simulink model "top_model"  (R2016a)
settings: Solver=ode1  StartTime=0  StopTime=20  FixedStep=0.001  RelTol=1e-3
undefined symbols (not defined in the file): env, veh_tyr, veh_veh_sx_0, veh_veh_vx_0
settings Model: Creator=The MathWorks, Inc.  LastModifiedBy=Renata
settings SolverCC: MaxOrder=3
settings DataIOCC: LimitDataPoints=on
settings DebuggingCC: AllowSymbolicDim=off
settings ModelReferenceCC: PropagateSignalLabelsOutOfModel=off
settings GRTTargetCC: GeneratePreprocessorConditionals=Use local settings

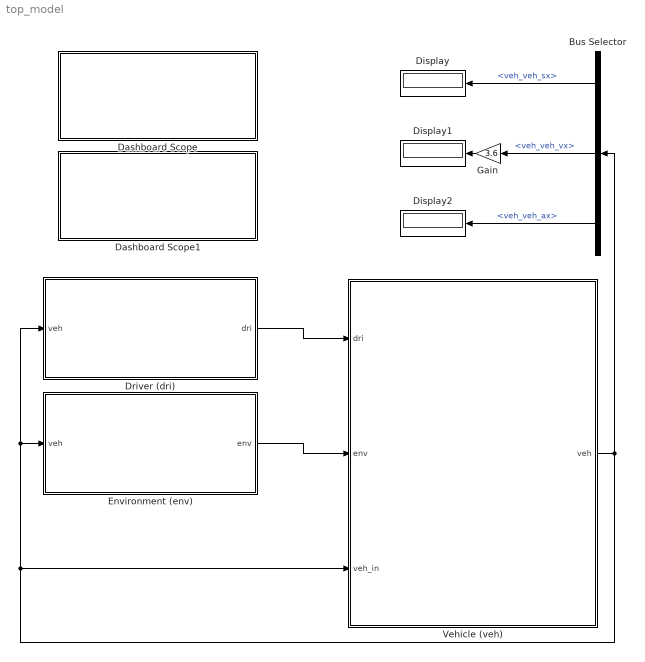
== system top_model ==
  Bus Selector : BusSelector  OutputSignals=veh_veh.veh_veh_sx,veh_veh.veh_veh_vx,veh_veh.veh_veh_ax
  Dashboard Scope : Subsystem  DialogController=hmiCreateDDGDialog  IsWebBlock=on  mask(MWDashboardBlock){webBlockId=2edd3ace-788d-40da-b228-b60fa6116b31, webBlockType=sdiscope, ShowInitialText=on, HMISrcModelName=top_model}
      mask prompts: webBlockId "WebBlock Id"; webBlockType "WebBlock Type"; HMISrcModelName "Source Model"
      mask Help: helpview([docroot '/mapfiles/simulink.map'], 'hmi_scope')
      mask Display:
      | if strcmp(get_param(bdroot(gcb),'BlockDiagramType'), 'library')
      |     image([(matlabroot) '/toolbox/simulink/hmi/icons/DashboardScope.png']);
      | end
  Dashboard Scope1 : Subsystem  DialogController=hmiCreateDDGDialog  IsWebBlock=on  mask(MWDashboardBlock){webBlockId=645ad2c4-08cc-4e51-8054-379eba2c8f07, webBlockType=sdiscope, ShowInitialText=on, HMISrcModelName=top_model}
      mask prompts: webBlockId "WebBlock Id"; webBlockType "WebBlock Type"; HMISrcModelName "Source Model"
      mask Help: helpview([docroot '/mapfiles/simulink.map'], 'hmi_scope')
      mask Display:
      | if strcmp(get_param(bdroot(gcb),'BlockDiagramType'), 'library')
      |     image([(matlabroot) '/toolbox/simulink/hmi/icons/DashboardScope.png']);
      | end
  Display : Display
  Display1 : Display
  Display2 : Display
  Driver (dri) : Subsystem  VariantControl=Variant
  Environment (env) : Subsystem
  Gain : Gain  Gain=3.6
  Vehicle (veh) : Subsystem
  wires:
  Driver (dri)/1(dri) -> Vehicle (veh)/1(dri)
  Environment (env)/1(env) -> Vehicle (veh)/2(env)
  Vehicle (veh)/1(veh) -> Bus Selector/1, Driver (dri)/1(veh), Environment (env)/1(veh), Vehicle (veh)/3(veh_in)
  Bus Selector/1 -> Display/1  "<veh_veh_sx>"
  Bus Selector/2 -> Gain/1  "<veh_veh_vx>"
  Bus Selector/3 -> Display2/1  "<veh_veh_ax>"
  Gain/1 -> Display1/1

== system top_model/Dashboard Scope ==

== system top_model/Dashboard Scope1 ==

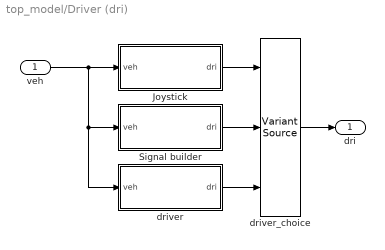
== system top_model/Driver (dri) ==
  veh : Inport
  Joystick : Subsystem  VariantControl=Variant
  Signal builder : Subsystem  VariantControl=Variant
  driver : Subsystem  VariantControl=Variant
  driver_choice : VariantSource  ShowConditionOnBlock=on
  dri : Outport
  wires:
  Signal builder/1(dri) -> driver_choice/2
  driver/1(dri) -> driver_choice/3
  Joystick/1(dri) -> driver_choice/1
  driver_choice/1 -> dri/1
  veh/1 -> driver/1(veh), Signal builder/1(veh), Joystick/1(veh)

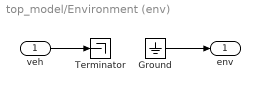
== system top_model/Environment (env) ==
  veh : Inport
  Ground : Ground
  Terminator : Terminator
  env : Outport
  wires:
  veh/1 -> Terminator/1
  Ground/1 -> env/1

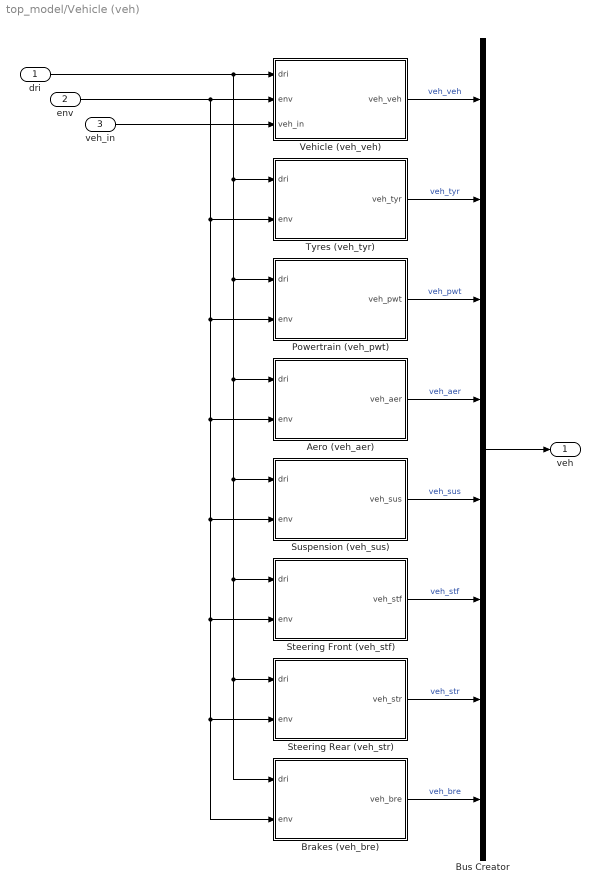
== system top_model/Vehicle (veh) ==
  dri : Inport
  env : Inport  Port=2
  veh_in : Inport  Port=3
  Aero (veh_aer) : Subsystem
  Brakes (veh_bre) : Subsystem
  Bus Creator : BusCreator  Inputs=8
  Powertrain (veh_pwt) : Subsystem
  Steering Front (veh_stf) : Subsystem
  Steering Rear (veh_str) : Subsystem
  Suspension (veh_sus) : Subsystem
  Tyres (veh_tyr) : Subsystem
  Vehicle (veh_veh) : Subsystem
  veh : Outport
  wires:
  Brakes (veh_bre)/1(veh_bre) -> Bus Creator/8  "veh_bre"
  Steering Rear (veh_str)/1(veh_str) -> Bus Creator/7  "veh_str"
  Steering Front (veh_stf)/1(veh_stf) -> Bus Creator/6  "veh_stf"
  Suspension (veh_sus)/1(veh_sus) -> Bus Creator/5  "veh_sus"
  Aero (veh_aer)/1(veh_aer) -> Bus Creator/4  "veh_aer"
  Powertrain (veh_pwt)/1(veh_pwt) -> Bus Creator/3  "veh_pwt"
  Tyres (veh_tyr)/1(veh_tyr) -> Bus Creator/2  "veh_tyr"
  Vehicle (veh_veh)/1(veh_veh) -> Bus Creator/1  "veh_veh"
  Bus Creator/1 -> veh/1
  dri/1 -> Brakes (veh_bre)/1(dri), Steering Rear (veh_str)/1(dri), Steering Front (veh_stf)/1(dri), Suspension (veh_sus)/1(dri), Aero (veh_aer)/1(dri), Powertrain (veh_pwt)/1(dri), Tyres (veh_tyr)/1(dri), Vehicle (veh_veh)/1(dri)
  env/1 -> Brakes (veh_bre)/2(env), Steering Rear (veh_str)/2(env), Steering Front (veh_stf)/2(env), Suspension (veh_sus)/2(env), Aero (veh_aer)/2(env), Powertrain (veh_pwt)/2(env), Tyres (veh_tyr)/2(env), Vehicle (veh_veh)/2(env)
  veh_in/1 -> Vehicle (veh_veh)/3(veh_in)

== system top_model/Driver (dri)/Joystick ==
  veh : Inport
  Ground : Ground
  Terminator : Terminator
  dri : Outport
  wires:
  veh/1 -> Terminator/1
  Ground/1 -> dri/1

== system top_model/Driver (dri)/Signal builder ==
  veh : Inport
  Ground : Ground
  Terminator : Terminator
  dri : Outport
  wires:
  veh/1 -> Terminator/1
  Ground/1 -> dri/1

== system top_model/Driver (dri)/driver ==
  veh : Inport
  Ground : Ground
  Terminator : Terminator
  dri : Outport
  wires:
  veh/1 -> Terminator/1
  Ground/1 -> dri/1

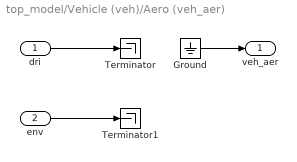
== system top_model/Vehicle (veh)/Aero (veh_aer) ==
  dri : Inport
  env : Inport  Port=2
  Ground : Ground
  Terminator : Terminator
  Terminator1 : Terminator
  veh_aer : Outport
  wires:
  dri/1 -> Terminator/1
  env/1 -> Terminator1/1
  Ground/1 -> veh_aer/1

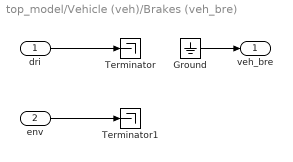
== system top_model/Vehicle (veh)/Brakes (veh_bre) ==
  dri : Inport
  env : Inport  Port=2
  Ground : Ground
  Terminator : Terminator
  Terminator1 : Terminator
  veh_bre : Outport
  wires:
  dri/1 -> Terminator/1
  env/1 -> Terminator1/1
  Ground/1 -> veh_bre/1

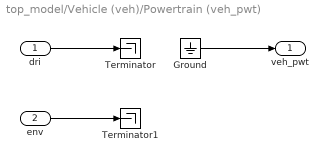
== system top_model/Vehicle (veh)/Powertrain (veh_pwt) ==
  dri : Inport
  env : Inport  Port=2
  Ground : Ground
  Terminator : Terminator
  Terminator1 : Terminator
  veh_pwt : Outport
  wires:
  dri/1 -> Terminator/1
  env/1 -> Terminator1/1
  Ground/1 -> veh_pwt/1

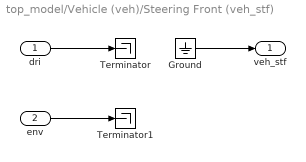
== system top_model/Vehicle (veh)/Steering Front (veh_stf) ==
  dri : Inport
  env : Inport  Port=2
  Ground : Ground
  Terminator : Terminator
  Terminator1 : Terminator
  veh_stf : Outport
  wires:
  dri/1 -> Terminator/1
  env/1 -> Terminator1/1
  Ground/1 -> veh_stf/1

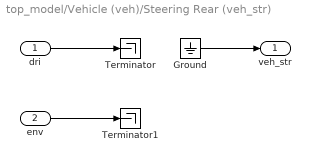
== system top_model/Vehicle (veh)/Steering Rear (veh_str) ==
  dri : Inport
  env : Inport  Port=2
  Ground : Ground
  Terminator : Terminator
  Terminator1 : Terminator
  veh_str : Outport
  wires:
  dri/1 -> Terminator/1
  env/1 -> Terminator1/1
  Ground/1 -> veh_str/1

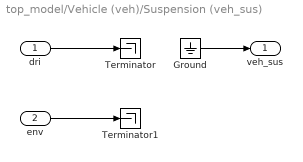
== system top_model/Vehicle (veh)/Suspension (veh_sus) ==
  dri : Inport
  env : Inport  Port=2
  Ground : Ground
  Terminator : Terminator
  Terminator1 : Terminator
  veh_sus : Outport
  wires:
  dri/1 -> Terminator/1
  env/1 -> Terminator1/1
  Ground/1 -> veh_sus/1

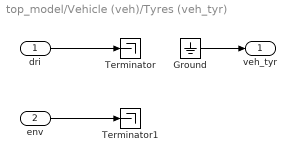
== system top_model/Vehicle (veh)/Tyres (veh_tyr) ==
  dri : Inport
  env : Inport  Port=2
  Ground : Ground
  Terminator : Terminator
  Terminator1 : Terminator
  veh_tyr : Outport
  wires:
  Ground/1 -> veh_tyr/1
  dri/1 -> Terminator/1
  env/1 -> Terminator1/1

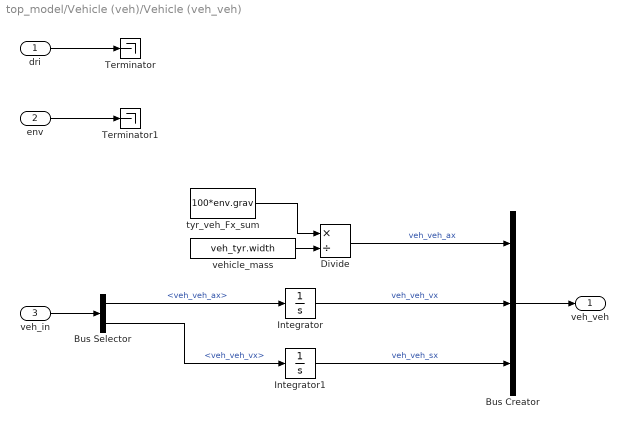
== system top_model/Vehicle (veh)/Vehicle (veh_veh) ==
  dri : Inport
  env : Inport  Port=2
  veh_in : Inport  Port=3
  Bus Creator : BusCreator  Inputs=3
  Bus Selector : BusSelector  OutputSignals=veh_veh.veh_veh_ax,veh_veh.veh_veh_vx
  Divide : Product  Inputs=*/  SaturateOnIntegerOverflow=on  RndMeth=Zero
  Integrator : Integrator  InitialCondition=veh_veh_vx_0
  Integrator1 : Integrator  InitialCondition=veh_veh_sx_0
  Terminator : Terminator
  Terminator1 : Terminator
  "tyr_veh_Fx_sum " : Constant  Value=100*env.grav
  vehicle_mass : Constant  Value=veh_tyr.width
  veh_veh : Outport
  wires:
  dri/1 -> Terminator/1
  env/1 -> Terminator1/1
  Bus Creator/1 -> veh_veh/1
  vehicle_mass/1 -> Divide/2
  "tyr_veh_Fx_sum "/1 -> Divide/1
  Divide/1 -> Bus Creator/1  "veh_veh_ax"
  veh_in/1 -> Bus Selector/1
  Bus Selector/1 -> Integrator/1  "<veh_veh_ax>"
  Integrator/1 -> Bus Creator/2  "veh_veh_vx"
  Integrator1/1 -> Bus Creator/3  "veh_veh_sx"
  Bus Selector/2 -> Integrator1/1  "<veh_veh_vx>"
